simulink subsystem "LimitedSlipDifferential"  (R2024b)
settings: Solver=VariableStepAuto  StartTime=0.0  StopTime=10.0  RelTol=1e-3
libraries: autolibshareddiff x1
settings Model: Creator=The MathWorks, Inc.  LastModifiedBy=The MathWorks, Inc.
settings RTWCC: GPUComputeCapability=3.5

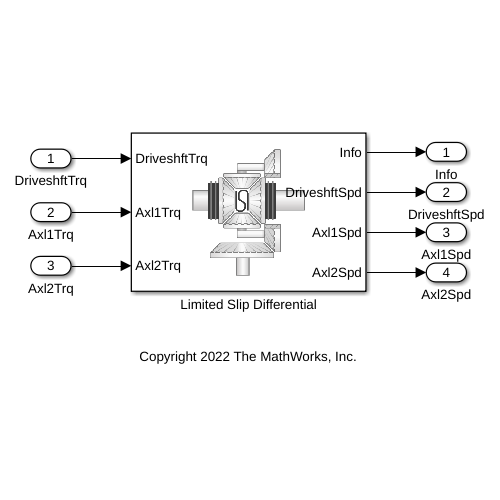
[thumbnail: Simulink's stored preview of the top-level diagram]
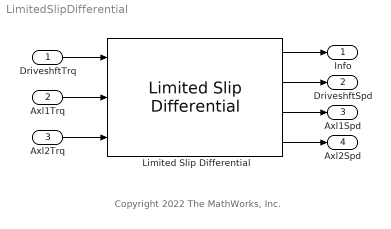
== system LimitedSlipDifferential ==
  note: Copyright 2022 The MathWorks, Inc.
  DriveshftTrq : Inport
  Axl1Trq : Inport  Port=2
  Axl2Trq : Inport  Port=3
  Limited Slip Differential : autolibshareddiff/Limited Slip Differential  VariantControl=Limited Slip Differential  DiffEffModelPopup=Constant  InterpMethod=Linear point-slope  extTamb=off  shaftSwitchMask=To the left of center-line  Ndiff=PlntDiffrntlRatio  Jd=PlntDiffrntlCarrInertia  bd=PlntDiffrntlCarrDamp  Jw1=PlntDiffrntlAxl1Inertia  bw1=PlntDiffrntlAxl1Damp  Jw2=PlntDiffrntlAxl2Inertia  bw2=PlntDiffrntlAxl2Damp  omegaw1o=PlntDiffrntlAxl1InitVel  omegaw2o=PlntDiffrntlAxl2InitVel  eta=PlntDiffrntlEff  eta_tbl=PlntDiffrntlEffTbl  Trq_bpts=PlntDiffrntlEffTrqBpt  omega_bpts=PlntDiffrntlEffSpdBpt  Temp_bpts=PlntDiffrntlEffTempBpt  Tamb=EnvAirTemp  couplingType=Pre-loaded ideal clutch  Ndisks=PlntDiffrntlCltchNumDisk  Reff=PlntDiffrntlCltchRadius  Fc=PlntDiffrntlCltchPreloadForce  muc=PlntDiffrntlCltchFricVect  dw=PlntDiffrntlCltchSpdVect  Tdw=PlntDiffrntlCltchTrqSlipSpdVect  dwT=PlntDiffrntlCltchSlipSpdVect  TTin=PlntDiffrntlCltchTrqInTrqVect  Tin=PlntDiffrntlCltchInTrqVect  tauC=PlntDiffrntlCltchCplngTimeCnst  IdealInterpMethod=Linear point-slope  IdealExtrapMethod=Linear  TdwInterpMethod=Flat  TdwExtrapMethod=Clip  TTinInterpMethod=Flat  TTinExtrapMethod=Clip  maxAbsSpd=5e3  aMode=6
  Info : Outport
  DriveshftSpd : Outport  Port=2
  Axl1Spd : Outport  Port=3
  Axl2Spd : Outport  Port=4
  wires:
  Limited Slip Differential/1 -> Info/1
  Limited Slip Differential/2 -> DriveshftSpd/1
  Limited Slip Differential/3 -> Axl1Spd/1
  Limited Slip Differential/4 -> Axl2Spd/1
  DriveshftTrq/1 -> Limited Slip Differential/1
  Axl1Trq/1 -> Limited Slip Differential/2
  Axl2Trq/1 -> Limited Slip Differential/3
